simulink model "digital_transmission"  (R2021a)
settings: Solver=VariableStepAuto  StartTime=0.0  StopTime=0.1  MaxStep=0.00001  MinStep=0.00000001  RelTol=1e-3
libraries: commutil2 x8, dspquant2 x8, dsparch4 x4, dspsigops x4, commdigbbndam3 x2
settings Model: Creator=Shakib  LastModifiedBy=mdnae
settings SolverCC: AlgebraicLoopSolver=TrustRegion
settings DataIOCC: ReturnWorkspaceOutputs=off
settings DebuggingCC: SFMachineParentedDataDiag=warning  ArithmeticOperatorsInVariantConditions=warning
settings SFSimCC: SimUseLocalCustomCode=off  CustomCodeUndefinedFunction=UseInterfaceOnly
settings RTWCC: RTWUseLocalCustomCode=off

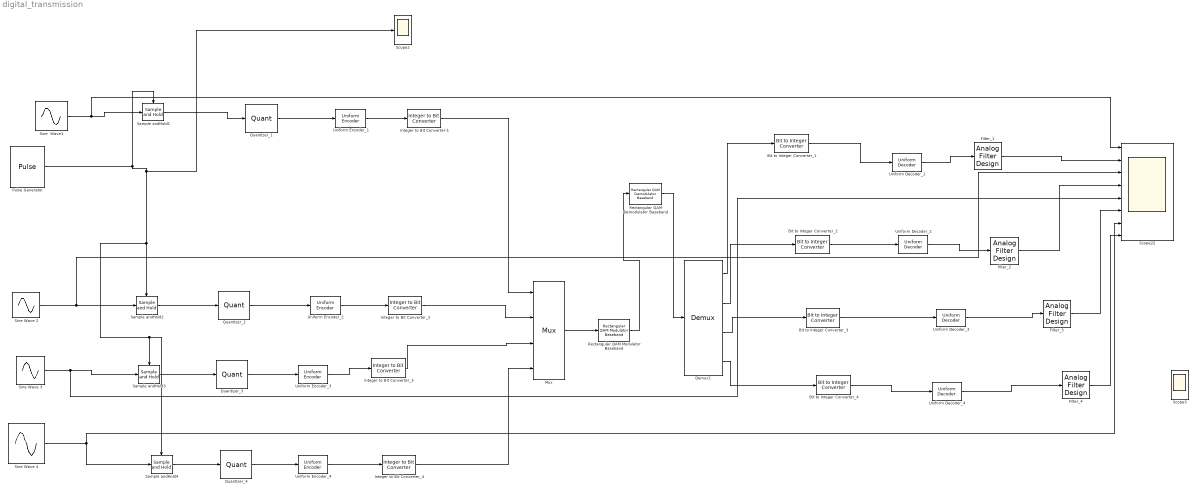
== system digital_transmission ==
  Bit to Integer Converter_{1..4} (4 alike) : commutil2/Bit to Integer Converter  nbits=4  bitOrder=MSB first  signedOutputValues=Signed  outDtype=Inherit via internal rule  outDtypeSigned=int8
  Demux1 : Demux
  Filter_1 : dsparch4/Analog Filter Design  method=Butterworth  filttype=Lowpass  N=8  Wlo=2*pi*5000  Whi=80  Rp=2  Rs=40
  Filter_3 : dsparch4/Analog Filter Design  method=Butterworth  filttype=Lowpass  N=8  Wlo=2*pi*8000  Whi=80  Rp=2  Rs=40
  Filter_4 : dsparch4/Analog Filter Design  method=Butterworth  filttype=Lowpass  N=8  Wlo=2*pi*3000  Whi=80  Rp=2  Rs=40
  Integer to Bit Converter-1 : commutil2/Integer to Bit Converter  nbits=4  signedInputValues=Signed  bitOrder=MSB first  outDtype=Inherit via internal rule
  Integer to Bit Converter_2 : commutil2/Integer to Bit Converter  nbits=4  signedInputValues=Signed  bitOrder=MSB first  outDtype=Inherit via internal rule
  Integer to Bit Converter_3 : commutil2/Integer to Bit Converter  nbits=4  signedInputValues=Signed  bitOrder=MSB first  outDtype=Inherit via internal rule
  Integer to Bit Converter_4 : commutil2/Integer to Bit Converter  nbits=4  signedInputValues=Signed  bitOrder=MSB first  outDtype=Inherit via internal rule
  Mux : Mux
  Pulse Generator : DiscretePulseGenerator  PulseType=Time based  Period=1/48000  PulseWidth=50
  Quantizer_{1..4} (4 alike) : Quantizer  QuantizationInterval=0.25
  Rectangular QAM Demodulator Baseband : commdigbbndam3/Rectangular QAM Demodulator Baseband  M=16  OutType=Bit  DecType=Hard decision  VarSource=Dialog  Variance=1  Dec=Gray  Mapping=[0:15]  PowType=Min. distance between symbols  MinDist=2  AvgPow=1  PeakPow=1  Ph=0  outDtype1=Inherit via internal rule  outDtype2=Inherit via internal rule  derotateFactorWordLen=16  derotateFactorDataTypeStr=Inherit: Same word length as input  derotateFactorLastDataTypeStr=Inherit: Same word length as input  denormFactorWordLen=16  denormFactorDataTypeStr=Inherit: Same word length as input  denormFactorLastDataTypeStr=Inherit: Same word length as input  prodOutWordLen=32  prodOutOverflowMode=Wrap  prodOutRoundingMode=Floor  prodOutOvFlMode=off  prodOutOvFlModeLastStrValue=off  sumWordLen=32
  Rectangular QAM Modulator Baseband : commdigbbndam3/Rectangular QAM Modulator Baseband  M=16  InType=Bit  Enc=Gray  Mapping=[0:15]  PowType=Min. distance between symbols  MinDist=2  AvgPow=1  PeakPow=1  Ph=0  outDtype=double  outWordLen=16  outUDDataType=sfix(16)  outFracLenMode=Best precision  outFracLen=15  outDataTypeStr=double  outLastDataTypeStr=double
  Sample andHold{1..4} (4 alike) : dspsigops/Sample and Hold  trig=Rising edge  initCond=0  latchinput=off
  Scope2 : Scope
  Scope22 : Scope  NumInputPorts=8
  Scope3 : Scope
  Sine  Wave1 : Sin  Frequency=2*pi*5000  Phase=pi/2  SampleTime=0
  Sine Wave 2 : Sin  Amplitude=2  Frequency=2*pi*8000  Phase=pi/2  SampleTime=0
  Sine Wave 3 : Sin  Amplitude=3  Frequency=2*pi*8000  Phase=pi/2  SampleTime=0
  Sine Wave 4 : Sin  Amplitude=4  Frequency=2*pi*3000  Phase=pi/2  SampleTime=0
  Uniform Decoder_1 : dspquant2/Uniform Decoder  peak=3.5  bits=3  overflowMode=Saturate  otype=Double
      settings: SourceProductBaseCode=DS
  Uniform Decoder_2 : dspquant2/Uniform Decoder  peak=4  bits=4  overflowMode=Saturate  otype=Double
      settings: SourceProductBaseCode=DS
  Uniform Decoder_3 : dspquant2/Uniform Decoder  peak=3  bits=4  overflowMode=Saturate  otype=Double
      settings: SourceProductBaseCode=DS
  Uniform Decoder_4 : dspquant2/Uniform Decoder  peak=3  bits=4  overflowMode=Saturate  otype=Double
      settings: SourceProductBaseCode=DS
  Uniform Encoder_1 : dspquant2/Uniform Encoder  peak=3.5  bits=4  otype=Signed integer
  Uniform Encoder_2 : dspquant2/Uniform Encoder  peak=1.5  bits=4  otype=Signed integer
  Uniform Encoder_3 : dspquant2/Uniform Encoder  peak=1.5  bits=4  otype=Signed integer
  Uniform Encoder_4 : dspquant2/Uniform Encoder  peak=1.5  bits=4  otype=Signed integer
  filter_2 : dsparch4/Analog Filter Design  method=Butterworth  filttype=Lowpass  N=8  Wlo=2*pi*8000  Whi=80  Rp=2  Rs=40
  wires:
  Uniform Encoder_1/1 -> Integer to Bit Converter-1/1
  Sample andHold1/1 -> Quantizer_1/1
  Sine  Wave1/1 -> Scope22/1, Sample andHold1/1
  Uniform Decoder_1/1 -> Filter_1/1
  Filter_1/1 -> Scope22/2
  Quantizer_1/1 -> Uniform Encoder_1/1
  Bit to Integer Converter_1/1 -> Uniform Decoder_1/1
  Rectangular QAM Modulator Baseband/1 -> Rectangular QAM Demodulator Baseband/1
  Sine Wave 2/1 -> Scope22/3, Sample andHold2/1
  Sine Wave 3/1 -> Scope22/5, Sample andHold3/1
  Sine Wave 4/1 -> Scope22/7, Sample andHold4/1
  Sample andHold3/1 -> Quantizer_3/1
  Sample andHold2/1 -> Quantizer_2/1
  Sample andHold4/1 -> Quantizer_4/1
  Quantizer_2/1 -> Uniform Encoder_2/1
  Quantizer_3/1 -> Uniform Encoder_3/1
  Quantizer_4/1 -> Uniform Encoder_4/1
  Uniform Encoder_2/1 -> Integer to Bit Converter_2/1
  Uniform Encoder_3/1 -> Integer to Bit Converter_3/1
  Uniform Encoder_4/1 -> Integer to Bit Converter_4/1
  Pulse Generator/1 -> Scope2/1, Sample andHold3/Trigger, Sample andHold4/Trigger, Sample andHold2/Trigger, Sample andHold1/Trigger
  Integer to Bit Converter-1/1 -> Mux/1
  Integer to Bit Converter_2/1 -> Mux/2
  Integer to Bit Converter_3/1 -> Mux/3
  Integer to Bit Converter_4/1 -> Mux/4
  Mux/1 -> Rectangular QAM Modulator Baseband/1
  Rectangular QAM Demodulator Baseband/1 -> Demux1/1
  Uniform Decoder_2/1 -> filter_2/1
  Bit to Integer Converter_2/1 -> Uniform Decoder_2/1
  Uniform Decoder_3/1 -> Filter_3/1
  Bit to Integer Converter_3/1 -> Uniform Decoder_3/1
  Uniform Decoder_4/1 -> Filter_4/1
  Bit to Integer Converter_4/1 -> Uniform Decoder_4/1
  Demux1/1 -> Bit to Integer Converter_1/1
  Demux1/2 -> Bit to Integer Converter_2/1
  Demux1/3 -> Bit to Integer Converter_3/1
  Demux1/4 -> Bit to Integer Converter_4/1
  Filter_3/1 -> Scope22/6
  filter_2/1 -> Scope22/4
  Filter_4/1 -> Scope22/8
